simulink model "AM_Demodulation"  (R2018b)
settings: Solver=VariableStepAuto  StartTime=0.0  StopTime=10.0  RelTol=1e-3
settings Model: Creator=sin  LastModifiedBy=sin

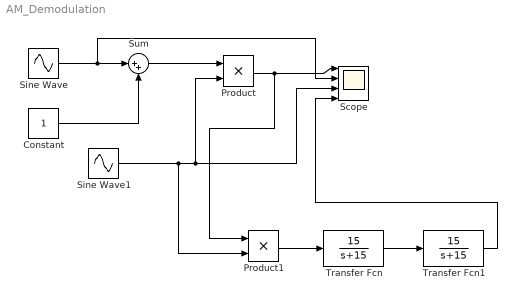
== system AM_Demodulation ==
  Constant : Constant
  Product : Product
  Product1 : Product
  Scope : Scope  NumInputPorts=4
  Sine Wave : Sin  Frequency=10  SampleTime=0
  Sine Wave1 : Sin  Frequency=50  SampleTime=0
  Sum : Sum  Inputs=|++
  Transfer Fcn : TransferFcn  Numerator=[15]  Denominator=[1 15]
  Transfer Fcn1 : TransferFcn  Numerator=[15]  Denominator=[1 15]
  wires:
  Product/1 -> Product1/1, Scope/1
  Sum/1 -> Product/1
  Sine Wave/1 -> Scope/2, Sum/1
  Sine Wave1/1 -> Product1/2, Scope/3, Product/2
  Constant/1 -> Sum/2
  Product1/1 -> Transfer Fcn/1
  Transfer Fcn/1 -> Transfer Fcn1/1
  Transfer Fcn1/1 -> Scope/4
